simulink model "GSM_sim_config_RC_RRC"  (Simulink 8.1)
settings: Solver=VariableStepDiscrete  StartTime=0.0  StopTime=simulationTime*10  RelTol=1e-3
values from neighbouring files (symbols this model uses):
  lengthOfSymbol = 64    [GSM_sim_config_RC_RRC_.m]
  sampleTime = 1    [GSM_sim_config_RC_RRC_.m]
libraries: commfilt2 x3, commchan3 x3, commdigbbndcpm2 x2, commdigbbndpm3 x1, commutil2 x1, dspsigops x1
settings Model: Creator=Philipp Fetzer  LastModifiedBy=mainster
settings OptimizationCC: ExpressionDepthLimit=128
settings DebuggingCC: StrictBusMsg=Warning

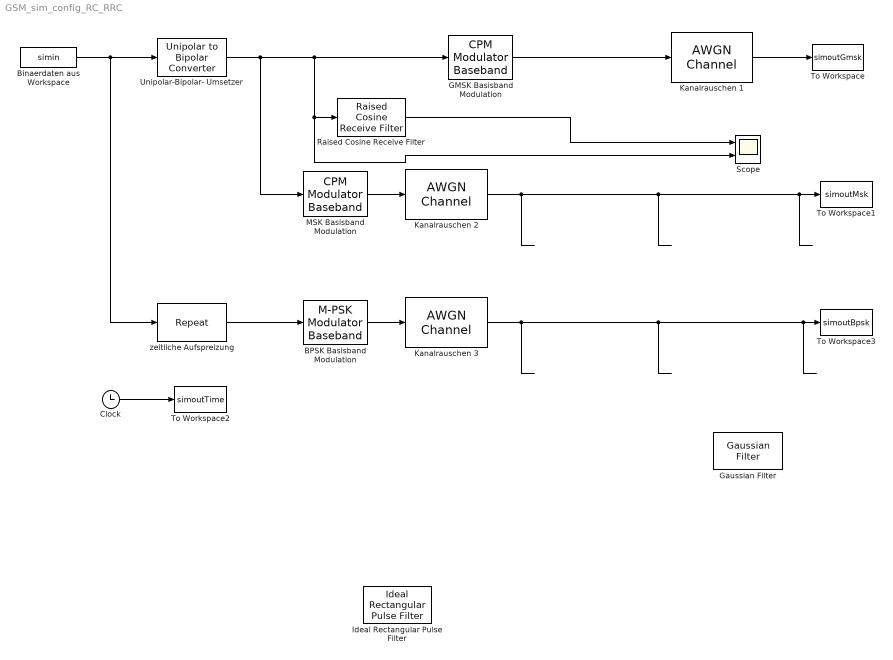
== system GSM_sim_config_RC_RRC ==
  BPSK Basisband Modulation : commdigbbndpm3/M-PSK Modulator Baseband  M=2  InType=Integer  Enc=Binary  Mapping=[0:2]  Ph=phaseOffset  outDtype=double  outWordLen=16  outUDDataType=sfix(16)  outFracLenMode=Best precision  outFracLen=15
  Binaerdaten aus Workspace : FromWorkspace  VariableName=simin  SampleTime=sampleTime
  Clock : Clock
  GMSK Basisband Modulation : commdigbbndcpm2/CPM Modulator Baseband  Mnum=2  inputType=Integer  mappingType=Binary  modIdx=.5  pulseShape=Gaussian  BT=.3  mainLobePulseLength=0.2  rollOff=0.2  pulseLength=4  preHistory=1  phaseOffset=phaseOffset  samplesPerSymbol=lengthOfSymbol  RateOptions=Inherit from input (this choice will be removed - see release notes)  outDataType=double
  Gaussian Filter : commfilt2/Gaussian Filter  N=8  BT=0.3  D=2  sampMode=Frame-based  normMode=Sum of coefficients  filterGain=1  checkCoeff=off  variableName=gaussFilt  launchFVT=off  roundingMode=Floor  overflowMode=off  InputProcessing=Columns as channels (frame based)
  Ideal Rectangular Pulse Filter : commfilt2/Ideal Rectangular Pulse Filter  pulseLen=8  pulseDelay=0  sampMode=Enforce single-rate processing  InputProcessing=Columns as channels (frame based)  normCheck=off  normMode=Sum of samples  filterGain=1  roundingMode=Floor  overflowMode=off
  Kanalrauschen 1 : commchan3/AWGN Channel  InputProcessing=Inherited (this choice will be removed - see release notes)  seed=67  noiseMode="Signal to noise ratio  (SNR)"  EbNodB=30  EsNodB=10  SNRdB=SNR  bitsPerSym=1  Ps=1  Tsym=1  variance=1
  Kanalrauschen 2 : commchan3/AWGN Channel  InputProcessing=Inherited (this choice will be removed - see release notes)  seed=67  noiseMode="Signal to noise ratio  (SNR)"  EbNodB=30  EsNodB=10  SNRdB=SNR  bitsPerSym=1  Ps=1  Tsym=1  variance=1
  Kanalrauschen 3 : commchan3/AWGN Channel  InputProcessing=Inherited (this choice will be removed - see release notes)  seed=67  noiseMode="Signal to noise ratio  (SNR)"  EbNodB=30  EsNodB=10  SNRdB=SNR  bitsPerSym=1  Ps=1  Tsym=1  variance=1
  MSK Basisband Modulation : commdigbbndcpm2/CPM Modulator Baseband  Mnum=2  inputType=Integer  mappingType=Binary  modIdx=0.5  pulseShape=Rectangular  BT=0.3  mainLobePulseLength=0.2  rollOff=0.2  pulseLength=1  preHistory=1  phaseOffset=phaseOffset  samplesPerSymbol=lengthOfSymbol  RateOptions=Inherit from input (this choice will be removed - see release notes)  outDataType=double
  Raised Cosine Receive Filter : commfilt2/Raised Cosine Receive Filter  filtType=Square root  N=8  D=5  R=0.5  sampMode=Mute  saveAsFlag=0  rateMode=None  downFactor=8  downOffset=0  framing=Enforce single-rate processing  InputProcessing=Columns as channels (frame based)  checkGain=Normalized  filterGain=1  checkCoeff=off  variableName=rcRxFilt  launchFVT=off  roundingMode=Floor  overflowMode=off
  Scope : Scope  NumInputPorts=2
      settings: ShowLegends=on  YMin=-5~-5  YMax=5~5
  To Workspace : ToWorkspace  VariableName=simoutGmsk  SampleTime=-1  SaveFormat=Structure
  To Workspace1 : ToWorkspace  VariableName=simoutMsk  SampleTime=-1  SaveFormat=Structure
  To Workspace2 : ToWorkspace  VariableName=simoutTime  SampleTime=-1  SaveFormat=Structure
  To Workspace3 : ToWorkspace  VariableName=simoutBpsk  SampleTime=-1  SaveFormat=Structure
  Unipolar-Bipolar- Umsetzer : commutil2/Unipolar to Bipolar Converter  M=2  polarity=Positive  dataType=Inherit via internal rule
  zeitliche Aufspreizung : dspsigops/Repeat  N=lengthOfSymbol  InputProcessing=Inherited (this choice will be removed - see release notes)  RateOptions=Allow multirate processing  ic=0  mode=Unused parameter value
  wires:
  MSK Basisband Modulation/1 -> Kanalrauschen 2/1
  Binaerdaten aus Workspace/1 -> Unipolar-Bipolar- Umsetzer/1, zeitliche Aufspreizung/1
  Clock/1 -> To Workspace2/1
  zeitliche Aufspreizung/1 -> BPSK Basisband Modulation/1
  BPSK Basisband Modulation/1 -> Kanalrauschen 3/1
  Kanalrauschen 2/1 -> To Workspace1/1
  Kanalrauschen 3/1 -> To Workspace3/1
  Unipolar-Bipolar- Umsetzer/1 -> Scope/2, Raised Cosine Receive Filter/1, GMSK Basisband Modulation/1, MSK Basisband Modulation/1
  Kanalrauschen 1/1 -> To Workspace/1
  GMSK Basisband Modulation/1 -> Kanalrauschen 1/1
  Raised Cosine Receive Filter/1 -> Scope/1
